simulink library "trl"  (Simulink 8.1)
settings: Solver=ode1  StartTime=0.0  StopTime=Inf  FixedStep=0.001  RelTol=1e-3
PostLoadFcn:
  | , if any(exist('dsrtsu_mdlpostloadfcn', 'file') == [2, 3, 6]), try dsrtsu_mdlpostloadfcn('Execute', bdroot); catch fprintf('Error in PostLoadFcn (dsrtsu_mdlpostloadfcn) for model "%s":\n %s\n', bdroot, lasterr); end, end,
undefined symbols (not defined in the file or in its folder): AACC_ACCVehSpd_mps, C_TICK_TIME_S, KACC_ACCMaxLatAccel_mps2, KACC_EngTqMaxMargin_Nm, KACC_EngTqMinMargin_Nm, KACC_LatAccelRollAvgInterval_s, KACC_LongAccelRollAvgInterval_s, MACC_ACCISOPosAcceleration_mps2
libraries: hcu_lib x4, idiada_lib x2
settings Model: DSRTSU_INTERNAL_RTI_VER=450  DSRTSU_INTERNAL_RTI_TYPE=rti1401  RTICANMMDATA=struct('GeneralSetupData',struct('modelroot','D:\ELN150201_TAIWAN\trunk\AdasDragon\software\sw_development\arch\app\acc','generalsettings',struct('filesettings',struct('destfolder',struct('Name','RTICANMM_FILES','Check',1),'buildfolder',struct('Name','.','Check',1),'AbsDestfolder',struct('Name','D:\ELN150201_TAIWAN\trunk\AdasDragon\software\sw_development\arch\app\acc\RTICANMM_FILES'),'AbsBuildfolder',struct('Name','D:\ELN150201_TAIWAN\trunk\AdasDragon\software\sw_development\arch\app\acc'))),'options',struct('addpaths',1,'rmpaths',1,'addtrcexclusion',logical(1),'cannavigator',struct('checkmonitoring',0),'show_usrtrc',0,'use_usrtrc',0),'advanced',struct('options',[1 1 1 1 1 1 1 1 1 1 1 1 1 1 1 1 1 1 1 1 1 1 1 1 1 1 1 1 1 1 1 1 1 1 1 1 1 1 1 1 1 1 1 1 1 1 1 1 1 1 1 1 1 1 1 1 1 1 1 1 1 1 1 1 1 1 1 1 1 1 1 1 1 1 1 1 1 1 1 1 1 1 1 1 1 1 1 1 1 1 1 1 1 1 1 1 1 1 1 1]),'MPSetup',{{}},'modelname','trl','block','trl'))  DSRTSU_INTERNAL_RTIFPGA=40  Creator=AT015411  LastModifiedBy=AT015555

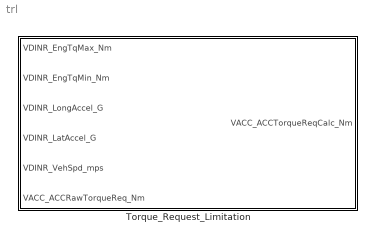
== system trl ==
  Torque_Request_Limitation : Subsystem

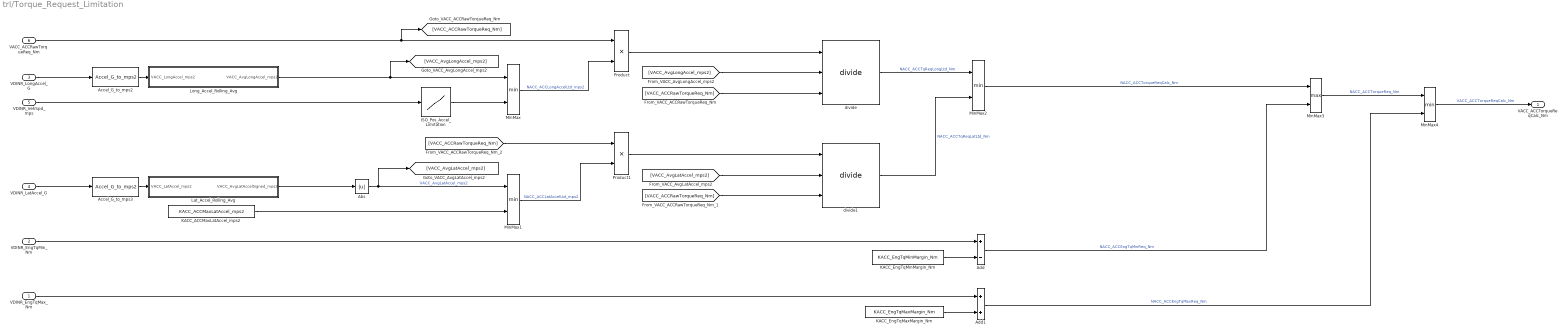
== system trl/Torque_Request_Limitation ==
  VDINR_EngTqMax_Nm : Inport
  VDINR_EngTqMin_Nm : Inport  Port=2
  VDINR_LongAccel_G : Inport  Port=3
  VDINR_LatAccel_G : Inport  Port=4
  VDINR_VehSpd_mps : Inport  Port=5
  VACC_ACCRawTorqueReq_Nm : Inport  Port=6
  Abs : Abs
  Accel_G_to_mps2 : idiada_lib/Accel_G_to_mps2
  Accel_G_to_mps3 : idiada_lib/Accel_G_to_mps2
  Add : Sum  Inputs=+-
  Add1 : Sum
  ISO_Pos_Accel_Limitation : Lookup_n-D  NumberOfTableDimensions=1  BreakpointsForDimension1=AACC_ACCVehSpd_mps  Table=MACC_ACCISOPosAcceleration_mps2  ExtrapMethod=Clip  UseLastTableValue=on  RndMeth=Simplest  InputSameDT=on
  KACC_ACCMaxLatAccel_mps2 : Constant  Value=KACC_ACCMaxLatAccel_mps2
  KACC_EngTqMaxMargin_Nm : Constant  Value=KACC_EngTqMaxMargin_Nm
  KACC_EngTqMinMargin_Nm : Constant  Value=KACC_EngTqMinMargin_Nm
  Lat_Accel_Rolling_Avg : Subsystem
  Long_Accel_Rolling_Avg : Subsystem
  MinMax{,1..2,4} (4 alike) : MinMax  Inputs=2
  MinMax3 : MinMax  Function=max  Inputs=2
  Product : Product
  Product1 : Product
  divide : hcu_lib/divide
  divide1 : hcu_lib/divide
  VACC_ACCTorqueReqCalc_Nm : Outport
  wires:
  MinMax4/1 -> VACC_ACCTorqueReqCalc_Nm/1  "VACC_ACCTorqueReqCalc_Nm"
  VDINR_EngTqMax_Nm/1 -> Add1/1
  MinMax3/1 -> MinMax4/1  "NACC_ACCTorqueReq_Nm"
  VDINR_EngTqMin_Nm/1 -> Add/1
  KACC_EngTqMinMargin_Nm/1 -> Add/2
  Add/1 -> MinMax3/2  "NACC_ACCEngTqMinReq_Nm"
  Add1/1 -> MinMax4/2  "NACC_ACCEngTqMaxReq_Nm"
  KACC_EngTqMaxMargin_Nm/1 -> Add1/2
  divide1/1 -> MinMax2/2  "NACC_ACCTqReqLatLtd_Nm"
  divide/1 -> MinMax2/1  "NACC_ACCTqReqLongLtd_Nm"
  [VACC_ACCRawTorqueReq_Nm] -> divide1/3
  [VACC_AvgLatAccel_mps2] -> divide1/2
  Product1/1 -> divide1/1
  [VACC_ACCRawTorqueReq_Nm] -> Product1/1
  MinMax1/1 -> Product1/2  "NACC_ACCLatAccelLtd_mps2"
  KACC_ACCMaxLatAccel_mps2/1 -> MinMax1/2
  Accel_G_to_mps3/1 -> Lat_Accel_Rolling_Avg/1(VACC_LatAccel_mps2)
  VDINR_LatAccel_G/1 -> Accel_G_to_mps3/1
  [VACC_ACCRawTorqueReq_Nm] -> divide/3
  Product/1 -> divide/1
  VACC_ACCRawTorqueReq_Nm/1 -> Product/1, [VACC_ACCRawTorqueReq_Nm]
  MinMax/1 -> Product/2  "NACC_ACCLongAccelLtd_mps2"
  [VACC_AvgLongAccel_mps2] -> divide/2
  ISO_Pos_Accel_Limitation/1 -> MinMax/2
  VDINR_VehSpd_mps/1 -> ISO_Pos_Accel_Limitation/1
  MinMax2/1 -> MinMax3/1  "NACC_ACCTorqueReqCalc_Nm"
  Accel_G_to_mps2/1 -> Long_Accel_Rolling_Avg/1(VACC_LongAccel_mps2)
  VDINR_LongAccel_G/1 -> Accel_G_to_mps2/1
  Long_Accel_Rolling_Avg/1(VACC_AvgLongAccel_mps2) -> [VACC_AvgLongAccel_mps2], MinMax/1
  Lat_Accel_Rolling_Avg/1(VACC_AvgLatAccelSigned_mps2) -> Abs/1
  Abs/1 -> MinMax1/1, [VACC_AvgLatAccel_mps2]  "VACC_AvgLatAccel_mps2"

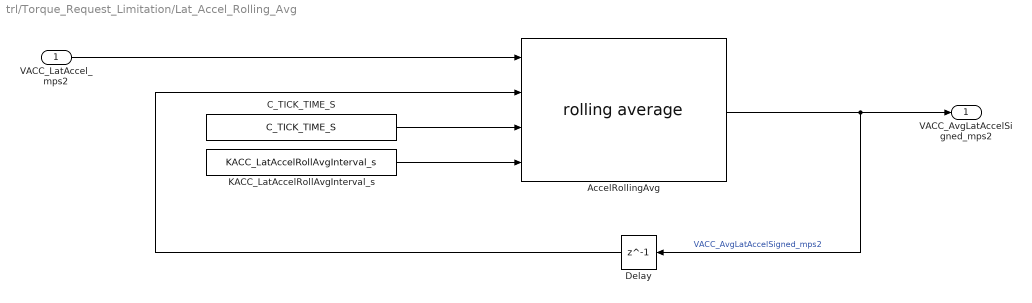
== system trl/Torque_Request_Limitation/Lat_Accel_Rolling_Avg ==
  VACC_LatAccel_mps2 : Inport
  AccelRollingAvg : hcu_lib/rolling average
  C_TICK_TIME_S : Constant  Value=C_TICK_TIME_S
  Delay : Delay  DelayLength=1
  KACC_LatAccelRollAvgInterval_s : Constant  Value=KACC_LatAccelRollAvgInterval_s
  VACC_AvgLatAccelSigned_mps2 : Outport
  wires:
  VACC_LatAccel_mps2/1 -> AccelRollingAvg/1
  C_TICK_TIME_S/1 -> AccelRollingAvg/3
  KACC_LatAccelRollAvgInterval_s/1 -> AccelRollingAvg/4
  AccelRollingAvg/1 -> Delay/1, VACC_AvgLatAccelSigned_mps2/1  "VACC_AvgLatAccelSigned_mps2"
  Delay/1 -> AccelRollingAvg/2

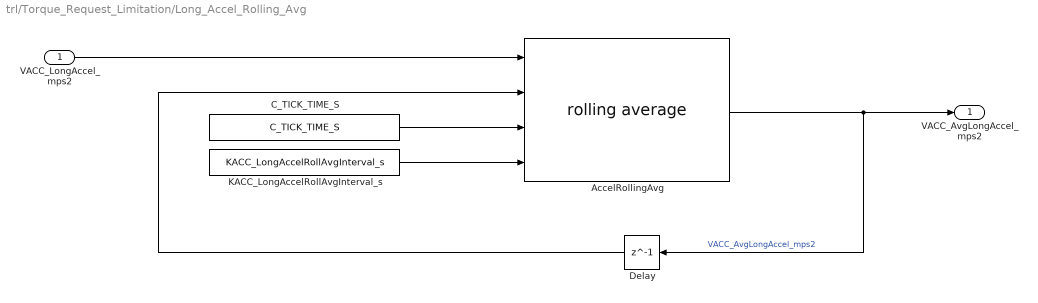
== system trl/Torque_Request_Limitation/Long_Accel_Rolling_Avg ==
  VACC_LongAccel_mps2 : Inport
  AccelRollingAvg : hcu_lib/rolling average
  C_TICK_TIME_S : Constant  Value=C_TICK_TIME_S
  Delay : Delay  DelayLength=1
  KACC_LongAccelRollAvgInterval_s : Constant  Value=KACC_LongAccelRollAvgInterval_s
  VACC_AvgLongAccel_mps2 : Outport
  wires:
  Delay/1 -> AccelRollingAvg/2
  AccelRollingAvg/1 -> VACC_AvgLongAccel_mps2/1, Delay/1  "VACC_AvgLongAccel_mps2"
  KACC_LongAccelRollAvgInterval_s/1 -> AccelRollingAvg/4
  C_TICK_TIME_S/1 -> AccelRollingAvg/3
  VACC_LongAccel_mps2/1 -> AccelRollingAvg/1
